simulink library "Lib_TestWatch"  (R2014b)
settings: Solver=ode45  StartTime=0.0  StopTime=10.0  RelTol=1e-3
settings Model: Creator=Ehang  LastModifiedBy=Ehang

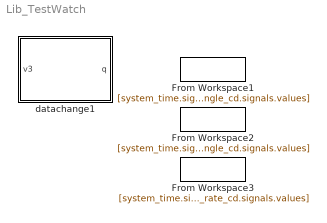
== system Lib_TestWatch ==
  From Workspace1 : FromWorkspace  VariableName=[system_time.signals.values,euler_roll_angle_cd.signals.values]  SampleTime=0
  From Workspace2 : FromWorkspace  VariableName=[system_time.signals.values,euler_pitch_angle_cd.signals.values]  SampleTime=0
  From Workspace3 : FromWorkspace  VariableName=[system_time.signals.values,euler_yaw_rate_cd.signals.values]  SampleTime=0
  datachange1 : MATLAB Function  TreatAsAtomicUnit=on

== matlab function Lib_TestWatch/datachange1 ==
  data: v3 input; q output
function q=datachange(v3)
q1=v3(1);
q2=v3(2);
q3=v3(3);
q=[q1;q2;q3];
